simulink model "ssc_vent_splitter_electrical_us_phs"  (R2020a)
settings: Solver=VariableStepAuto  StartTime=0.0  StopTime=10.0  RelTol=1e-3
model workspace: external: MAT-File /Users/jsolislemus/Documents/MATLAB/ssc.ventilator-splitter/Ventilator_Electrical_Parameters_SIUnits.mat (data not in the file)
values from neighbouring files (symbols this model uses):
  IE_ratio = 0.5    [Ventilator_Electrical_Parameters.mat]    (also in Ventilator_Electrical_Parameters_SIUnits.mat; setInitialParameters.m)
  R_D1 = 1    [Ventilator_Electrical_Parameters.mat]    (also in Ventilator_Electrical_Parameters_SIUnits.mat = 4000; setInitialParameters.m = 4000)
  R_D2 = 1    [Ventilator_Electrical_Parameters.mat]    (also in Ventilator_Electrical_Parameters_SIUnits.mat = 4000; setInitialParameters.m = 4000)
  R_E1 = 1    [Ventilator_Electrical_Parameters.mat]    (also in Ventilator_Electrical_Parameters_SIUnits.mat = 4000; setInitialParameters.m = 4000)
  R_E2 = 1    [Ventilator_Electrical_Parameters.mat]    (also in Ventilator_Electrical_Parameters_SIUnits.mat = 4000; setInitialParameters.m = 4000)
  R_ETT1 = 1961330    [Ventilator_Electrical_Parameters_SIUnits.mat]    (also in setInitialParameters.m)
  R_ETT2 = 1961330    [Ventilator_Electrical_Parameters_SIUnits.mat]    (also in setInitialParameters.m)
  R_L1 = 100    [Ventilator_Electrical_Parameters.mat]    (also in Ventilator_Electrical_Parameters_SIUnits.mat = 196133; setInitialParameters.m = 196133)
  R_L2 = 100    [Ventilator_Electrical_Parameters.mat]    (also in Ventilator_Electrical_Parameters_SIUnits.mat = 196133; setInitialParameters.m = 196133)
  R_U1 = 1    [Ventilator_Electrical_Parameters.mat]    (also in Ventilator_Electrical_Parameters_SIUnits.mat = 4000; setInitialParameters.m = 4000)
  R_U2 = 1    [Ventilator_Electrical_Parameters.mat]    (also in Ventilator_Electrical_Parameters_SIUnits.mat = 4000; setInitialParameters.m = 4000)
  RR = 15    [Ventilator_Electrical_Parameters.mat]    (also in Ventilator_Electrical_Parameters_SIUnits.mat; setInitialParameters.m; test_vent_pressure.m)
  v_M_exhale = 5    [Ventilator_Electrical_Parameters.mat]    (also in Ventilator_Electrical_Parameters_SIUnits.mat = 490)
  v_M_inhale = 20    [Ventilator_Electrical_Parameters.mat]    (also in Ventilator_Electrical_Parameters_SIUnits.mat = 1960; setInitialParameters.m = 1960)
libraries: fl_lib x32, nesl_utility x13
settings Model: Creator=jsolislemus  LastModifiedBy=jsolislemus

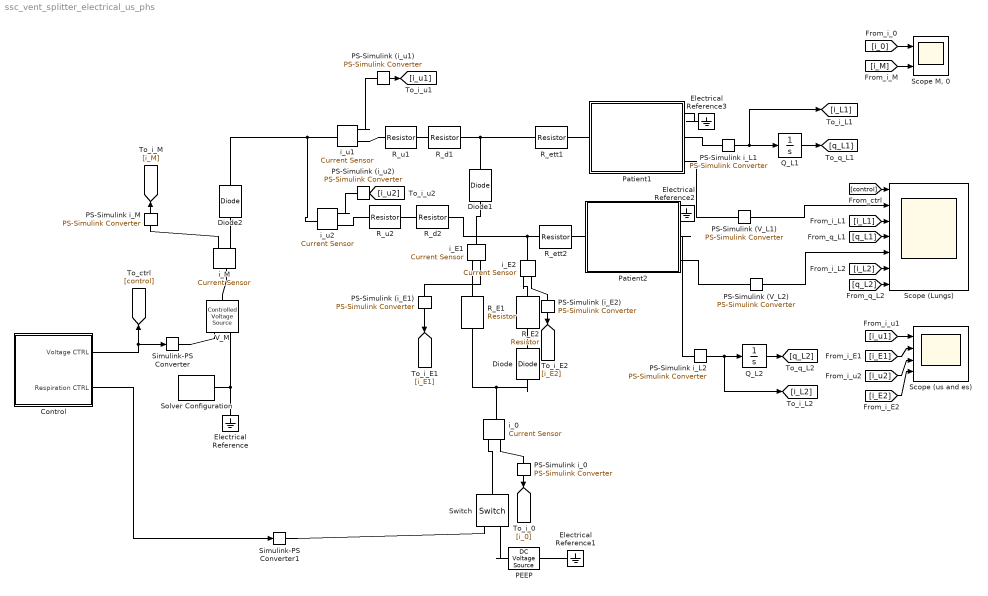
== system ssc_vent_splitter_electrical_us_phs ==
  Control : Subsystem
  Diode : fl_lib/Electrical/Electrical Elements/Diode  Vf=0.6 V  Ron=0.3 Ohm  Goff=1e-8 1/Ohm  i_specify=off  i_priority=None  i=0 A  i_nominal_specify=off  i_nominal_unit=A  i_nominal_value=1  v_specify=off  v_priority=None  v=0 V  v_nominal_specify=off  v_nominal_unit=V  v_nominal_value=1
  Diode1 : fl_lib/Electrical/Electrical Elements/Diode  Vf=0.6 V  Ron=0.3 Ohm  Goff=1e-8 1/Ohm  i_specify=off  i_priority=None  i=0 A  i_nominal_specify=off  i_nominal_unit=A  i_nominal_value=1  v_specify=off  v_priority=None  v=0 V  v_nominal_specify=off  v_nominal_unit=V  v_nominal_value=1
  Diode2 : fl_lib/Electrical/Electrical Elements/Diode  Vf=0.6 V  Ron=0.3 Ohm  Goff=1e-8 1/Ohm  i_specify=off  i_priority=None  i=0 A  i_nominal_specify=off  i_nominal_unit=A  i_nominal_value=1  v_specify=off  v_priority=None  v=0 V  v_nominal_specify=off  v_nominal_unit=V  v_nominal_value=1
  Electrical Reference{,1..3} (4 alike) : fl_lib/Electrical/Electrical Elements/Electrical Reference
  PEEP : fl_lib/Electrical/Electrical Sources/DC Voltage Source  v0=v_M_exhale V
  PS-Simulink (V_L1) : nesl_utility/PS-Simulink Converter  PhysicalDomain=network_engine_domain  SubClassName=ps_output  LeftPortType=input  RightPortType=output  PseudoPeriodic=off  Frequencies=[]  Unit=inherit  AffineConversion=off
  PS-Simulink (V_L2) : nesl_utility/PS-Simulink Converter  PhysicalDomain=network_engine_domain  SubClassName=ps_output  LeftPortType=input  RightPortType=output  PseudoPeriodic=off  Frequencies=[]  Unit=inherit  AffineConversion=off
  PS-Simulink (i_E1) : nesl_utility/PS-Simulink Converter  PhysicalDomain=network_engine_domain  SubClassName=ps_output  LeftPortType=input  RightPortType=output  PseudoPeriodic=off  Frequencies=[]  Unit=inherit  AffineConversion=off
  PS-Simulink (i_E2) : nesl_utility/PS-Simulink Converter  PhysicalDomain=network_engine_domain  SubClassName=ps_output  LeftPortType=input  RightPortType=output  PseudoPeriodic=off  Frequencies=[]  Unit=inherit  AffineConversion=off
  PS-Simulink (i_u1) : nesl_utility/PS-Simulink Converter  PhysicalDomain=network_engine_domain  SubClassName=ps_output  LeftPortType=input  RightPortType=output  PseudoPeriodic=off  Frequencies=[]  Unit=inherit  AffineConversion=off
  PS-Simulink (i_u2) : nesl_utility/PS-Simulink Converter  PhysicalDomain=network_engine_domain  SubClassName=ps_output  LeftPortType=input  RightPortType=output  PseudoPeriodic=off  Frequencies=[]  Unit=inherit  AffineConversion=off
  PS-Simulink i_0 : nesl_utility/PS-Simulink Converter  PhysicalDomain=network_engine_domain  SubClassName=ps_output  LeftPortType=input  RightPortType=output  PseudoPeriodic=off  Frequencies=[]  Unit=inherit  AffineConversion=off
  PS-Simulink i_L1 : nesl_utility/PS-Simulink Converter  PhysicalDomain=network_engine_domain  SubClassName=ps_output  LeftPortType=input  RightPortType=output  PseudoPeriodic=off  Frequencies=[]  Unit=inherit  AffineConversion=off
  PS-Simulink i_L2 : nesl_utility/PS-Simulink Converter  PhysicalDomain=network_engine_domain  SubClassName=ps_output  LeftPortType=input  RightPortType=output  PseudoPeriodic=off  Frequencies=[]  Unit=inherit  AffineConversion=off
  PS-Simulink i_M : nesl_utility/PS-Simulink Converter  PhysicalDomain=network_engine_domain  SubClassName=ps_output  LeftPortType=input  RightPortType=output  PseudoPeriodic=off  Frequencies=[]  Unit=inherit  AffineConversion=off
  Patient1 : Subsystem
  Patient2 : Subsystem
  Q_L1 : Integrator
  Q_L2 : Integrator
  R_E1 : fl_lib/Electrical/Electrical Elements/Resistor  R=R_E1 Ohm  i_specify=off  i_priority=None  i=0 A  i_nominal_specify=off  i_nominal_unit=A  i_nominal_value=1  v_specify=off  v_priority=None  v=0 V  v_nominal_specify=off  v_nominal_unit=V  v_nominal_value=1
  R_E2 : fl_lib/Electrical/Electrical Elements/Resistor  R=R_E2 Ohm  i_specify=off  i_priority=None  i=0 A  i_nominal_specify=off  i_nominal_unit=A  i_nominal_value=1  v_specify=off  v_priority=None  v=0 V  v_nominal_specify=off  v_nominal_unit=V  v_nominal_value=1
  R_d1 : fl_lib/Electrical/Electrical Elements/Resistor  R=R_D1 Ohm  i_specify=off  i_priority=None  i=0 A  i_nominal_specify=off  i_nominal_unit=A  i_nominal_value=1  v_specify=off  v_priority=None  v=0 V  v_nominal_specify=off  v_nominal_unit=V  v_nominal_value=1
  R_d2 : fl_lib/Electrical/Electrical Elements/Resistor  R=R_D2 Ohm  i_specify=off  i_priority=None  i=0 A  i_nominal_specify=off  i_nominal_unit=A  i_nominal_value=1  v_specify=off  v_priority=None  v=0 V  v_nominal_specify=off  v_nominal_unit=V  v_nominal_value=1
  R_ett1 : fl_lib/Electrical/Electrical Elements/Resistor  R=R_ETT1 Ohm  i_specify=off  i_priority=None  i=0 A  i_nominal_specify=off  i_nominal_unit=A  i_nominal_value=1  v_specify=off  v_priority=None  v=0 V  v_nominal_specify=off  v_nominal_unit=V  v_nominal_value=1
  R_ett2 : fl_lib/Electrical/Electrical Elements/Resistor  R=R_ETT2 Ohm  i_specify=off  i_priority=None  i=0 A  i_nominal_specify=off  i_nominal_unit=A  i_nominal_value=1  v_specify=off  v_priority=None  v=0 V  v_nominal_specify=off  v_nominal_unit=V  v_nominal_value=1
  R_u1 : fl_lib/Electrical/Electrical Elements/Resistor  R=R_U1 Ohm  i_specify=off  i_priority=None  i=0 A  i_nominal_specify=off  i_nominal_unit=A  i_nominal_value=1  v_specify=off  v_priority=None  v=0 V  v_nominal_specify=off  v_nominal_unit=V  v_nominal_value=1
  R_u2 : fl_lib/Electrical/Electrical Elements/Resistor  R=R_U2 Ohm  i_specify=off  i_priority=None  i=0 A  i_nominal_specify=off  i_nominal_unit=A  i_nominal_value=1  v_specify=off  v_priority=None  v=0 V  v_nominal_specify=off  v_nominal_unit=V  v_nominal_value=1
  Scope (Lungs) : Scope  NumInputPorts=7
  Scope (us and es) : Scope  NumInputPorts=4
  "Scope M, 0" : Scope  NumInputPorts=2
  Simulink-PS Converter : nesl_utility/Simulink-PS Converter  PhysicalDomain=network_engine_domain  SubClassName=ps_input  LeftPortType=input  RightPortType=output  PseudoPeriodic=off  Frequencies=[]  NoiseDistribution=none  NoiseParameters=[]  Unit=1  AffineConversion=off  FilteringAndDerivatives=provide  SimscapeFilterOrder=1  InputFilterTimeConstant=0.001  UdotUserProvided=0
  Simulink-PS Converter1 : nesl_utility/Simulink-PS Converter  PhysicalDomain=network_engine_domain  SubClassName=ps_input  LeftPortType=input  RightPortType=output  PseudoPeriodic=off  Frequencies=[]  NoiseDistribution=none  NoiseParameters=[]  Unit=1  AffineConversion=off  FilteringAndDerivatives=provide  SimscapeFilterOrder=1  InputFilterTimeConstant=0.001  UdotUserProvided=0
  Solver Configuration : nesl_utility/Solver Configuration  PhysicalDomain=network_engine_domain  SubClassName=solver  LeftPortType=input  RightPortType=generic  Tones=[]  Harmonics=[]  SimulateNoise=off  Profile=off  UseLocalSampling=off  EnableSwitchedLinearOptims=on  FrequencyDomain=off  UseCCode=off  RelTol=0.001  AbsTol=1e-06  MinStep=1e-09  ToWorkspace=off  RevertToSquareIcSolve=off  NumHomotopyIterations=100  PhasorMode=off  PhasorModeNumHarmonics=1  DoDC=off  ResidualTolerance=1e-09  UseLocalSolver=off  LocalSolverChoice=NE_BACKWARD_EULER_ADVANCER  LocalSolverSampleTime=0.001  DoFixedCost=off  MaxNonlinIter=3  MaxModeIter=2  LinearAlgebra=auto  EquationFormulation=NE_TIME_EF  DelaysMemoryBudget=1024  AutomaticFiltering=on  FilteringTimeConstant=0.001  PartitionStorageMethod=AS_NEEDED  PartitionMemoryBudget=1024  PartitionMethod=ROBUST
  Switch : fl_lib/Electrical/Electrical Elements/Switch  R_closed=0.01 Ohm  G_open=1e-8 1/Ohm  Threshold=0.5  i_specify=off  i_priority=None  i=0 A  i_nominal_specify=off  i_nominal_unit=A  i_nominal_value=1  v_specify=off  v_priority=None  v=0 V  v_nominal_specify=off  v_nominal_unit=V  v_nominal_value=1
  V_M : fl_lib/Electrical/Electrical Sources/Controlled Voltage Source
  i_0 : fl_lib/Electrical/Electrical Sensors/Current Sensor
  i_E1 : fl_lib/Electrical/Electrical Sensors/Current Sensor
  i_E2 : fl_lib/Electrical/Electrical Sensors/Current Sensor
  i_M : fl_lib/Electrical/Electrical Sensors/Current Sensor
  i_u1 : fl_lib/Electrical/Electrical Sensors/Current Sensor
  i_u2 : fl_lib/Electrical/Electrical Sensors/Current Sensor
  wires:
  PS-Simulink i_L1/1 -> [i_L1], Q_L1/1
  PS-Simulink i_L2/1 -> [i_L2], Q_L2/1
  Q_L1/1 -> [q_L1]
  Q_L2/1 -> [q_L2]
  PS-Simulink (i_u1)/1 -> [i_u1]
  [i_u1] -> Scope (us and es)/1
  [i_u2] -> Scope (us and es)/3
  PS-Simulink (i_u2)/1 -> [i_u2]
  [i_E1] -> Scope (us and es)/2
  [i_E2] -> Scope (us and es)/4
  PS-Simulink (i_E2)/1 -> [i_E2]
  [i_0] -> "Scope M, 0"/1
  PS-Simulink i_0/1 -> [i_0]
  PS-Simulink i_M/1 -> [i_M]
  [i_M] -> "Scope M, 0"/2
  PS-Simulink (i_E1)/1 -> [i_E1]
  [control] -> Scope (Lungs)/1
  [q_L2] -> Scope (Lungs)/7
  [i_L2] -> Scope (Lungs)/6
  [q_L1] -> Scope (Lungs)/4
  PS-Simulink (V_L1)/1 -> Scope (Lungs)/2
  PS-Simulink (V_L2)/1 -> Scope (Lungs)/5
  [i_L1] -> Scope (Lungs)/3
  Control/1(Voltage CTRL) -> [control], Simulink-PS Converter/1
  Control/2(Respiration CTRL) -> Simulink-PS Converter1/1
  connections:
  Simulink-PS Converter/RConn1 -- V_M/RConn1
  V_M/RConn2 -- Solver Configuration/RConn1 -- Electrical Reference/LConn1
  i_u1/LConn1 -- Diode2/RConn1 -- i_u2/LConn1
  R_d2/LConn1 -- R_u2/RConn1
  R_u1/RConn1 -- R_d1/LConn1
  Simulink-PS Converter1/RConn1 -- Switch/RConn1
  i_u1/RConn2 -- R_u1/LConn1
  i_u2/RConn2 -- R_u2/LConn1
  i_E2/RConn2 -- R_E2/LConn1
  i_M/LConn1 -- V_M/LConn1
  i_0/RConn2 -- Switch/LConn1
  i_u1/RConn1 -- PS-Simulink (i_u1)/LConn1
  i_u2/RConn1 -- PS-Simulink (i_u2)/LConn1
  i_0/RConn1 -- PS-Simulink i_0/LConn1
  i_E2/RConn1 -- PS-Simulink (i_E2)/LConn1
  i_E1/RConn1 -- PS-Simulink (i_E1)/LConn1
  i_M/RConn1 -- PS-Simulink i_M/LConn1
  Electrical Reference3/LConn1 -- Patient1/RConn1
  Patient1/RConn2 -- PS-Simulink i_L1/LConn1
  Patient1/RConn3 -- PS-Simulink (V_L1)/LConn1
  Electrical Reference2/LConn1 -- Patient2/RConn1
  Patient2/RConn3 -- PS-Simulink (V_L2)/LConn1
  Patient2/RConn2 -- PS-Simulink i_L2/LConn1
  R_E1/LConn1 -- i_E1/RConn2
  i_0/LConn1 -- R_E1/RConn1 -- Diode/RConn1
  R_ett1/RConn1 -- Patient1/LConn1
  R_ett1/LConn1 -- Diode1/LConn1 -- R_d1/RConn1
  R_ett2/LConn1 -- i_E2/LConn1 -- R_d2/RConn1
  R_ett2/RConn1 -- Patient2/LConn1
  Diode1/RConn1 -- i_E1/LConn1
  Diode/LConn1 -- R_E2/RConn1
  Diode2/LConn1 -- i_M/RConn2
  PEEP/LConn1 -- Switch/RConn2
  Electrical Reference1/LConn1 -- PEEP/RConn1

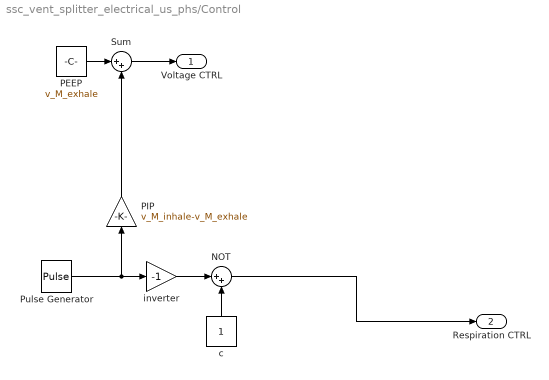
== system ssc_vent_splitter_electrical_us_phs/Control ==
  NOT : Sum  Inputs=|++
  PEEP : Constant  Value=v_M_exhale
  PIP : Gain  Gain=v_M_inhale-v_M_exhale
  Pulse Generator : DiscretePulseGenerator  PulseType=Time based  Period=60 / RR  PulseWidth=IE_ratio/(IE_ratio+1)*100
  Sum : Sum  Inputs=|++
  c : Constant
  inverter : Gain  Gain=-1
  Voltage CTRL : Outport
  Respiration CTRL : Outport  Port=2
  wires:
  NOT/1 -> Respiration CTRL/1
  Pulse Generator/1 -> inverter/1, PIP/1
  inverter/1 -> NOT/1
  Sum/1 -> Voltage CTRL/1
  PEEP/1 -> Sum/1
  PIP/1 -> Sum/2
  c/1 -> NOT/2

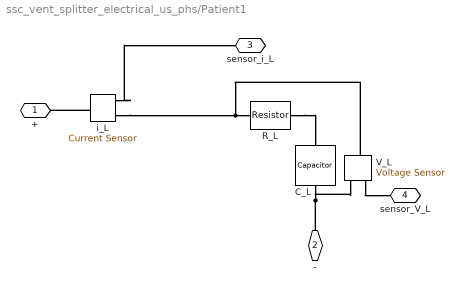
== system ssc_vent_splitter_electrical_us_phs/Patient1 ==
  C_L : fl_lib/Electrical/Electrical Elements/Capacitor  c=C_L1 F  r=1e-6 Ohm  g=0 1/Ohm  i_specify=off  i_priority=None  i=0 A  i_nominal_specify=off  i_nominal_unit=A  i_nominal_value=1  v_specify=off  v_priority=None  v=0 V  v_nominal_specify=off  v_nominal_unit=V  v_nominal_value=1  vc_specify=off  vc_priority=High  vc=0 V  vc_nominal_specify=off  vc_nominal_unit=V  vc_nominal_value=1
  R_L : fl_lib/Electrical/Electrical Elements/Resistor  R=R_L1 Ohm  i_specify=off  i_priority=None  i=0 A  i_nominal_specify=off  i_nominal_unit=A  i_nominal_value=1  v_specify=off  v_priority=None  v=0 V  v_nominal_specify=off  v_nominal_unit=V  v_nominal_value=1
  V_L : fl_lib/Electrical/Electrical Sensors/Voltage Sensor
  i_L : fl_lib/Electrical/Electrical Sensors/Current Sensor
  + : PMIOPort  Side=Left
  - : PMIOPort  Port=2  Side=Right
  sensor_i_L : PMIOPort  Port=3  Side=Right
  sensor_V_L : PMIOPort  Port=4  Side=Right
  connections:
  i_L/LConn1 -- +/RConn1
  C_L/RConn1 -- V_L/RConn2 -- -/RConn1
  i_L/RConn1 -- sensor_i_L/RConn1
  V_L/RConn1 -- sensor_V_L/RConn1
  R_L/RConn1 -- C_L/LConn1
  R_L/LConn1 -- i_L/RConn2 -- V_L/LConn1

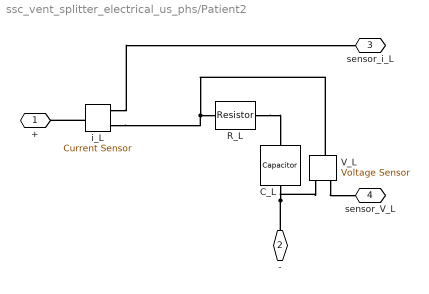
== system ssc_vent_splitter_electrical_us_phs/Patient2 ==
  C_L : fl_lib/Electrical/Electrical Elements/Capacitor  c=C_L2 F  r=1e-6 Ohm  g=0 1/Ohm  i_specify=off  i_priority=None  i=0 A  i_nominal_specify=off  i_nominal_unit=A  i_nominal_value=1  v_specify=off  v_priority=None  v=0 V  v_nominal_specify=off  v_nominal_unit=V  v_nominal_value=1  vc_specify=off  vc_priority=High  vc=0 V  vc_nominal_specify=off  vc_nominal_unit=V  vc_nominal_value=1
  R_L : fl_lib/Electrical/Electrical Elements/Resistor  R=R_L2 Ohm  i_specify=off  i_priority=None  i=0 A  i_nominal_specify=off  i_nominal_unit=A  i_nominal_value=1  v_specify=off  v_priority=None  v=0 V  v_nominal_specify=off  v_nominal_unit=V  v_nominal_value=1
  V_L : fl_lib/Electrical/Electrical Sensors/Voltage Sensor
  i_L : fl_lib/Electrical/Electrical Sensors/Current Sensor
  + : PMIOPort  Side=Left
  - : PMIOPort  Port=2  Side=Right
  sensor_i_L : PMIOPort  Port=3  Side=Right
  sensor_V_L : PMIOPort  Port=4  Side=Right
  connections:
  i_L/LConn1 -- +/RConn1
  V_L/RConn2 -- C_L/RConn1 -- -/RConn1
  i_L/RConn1 -- sensor_i_L/RConn1
  V_L/RConn1 -- sensor_V_L/RConn1
  R_L/RConn1 -- C_L/LConn1
  V_L/LConn1 -- i_L/RConn2 -- R_L/LConn1
